simulink model "Spartan2Serial"  (R2019a)
settings: Solver=FixedStepDiscrete  StartTime=0.0  StopTime=inf  FixedStep=0.01  RelTol=1e-3
undefined symbols (not defined in the file): serial
libraries: instrumentlib x2
settings Model: SimulationMode=accelerator  EnablePacing=on  Creator=manuk  LastModifiedBy=manuk
settings DataIOCC: SaveOutput=off  SignalLogging=off  DSMLogging=off  SaveTime=off  ReturnWorkspaceOutputs=off

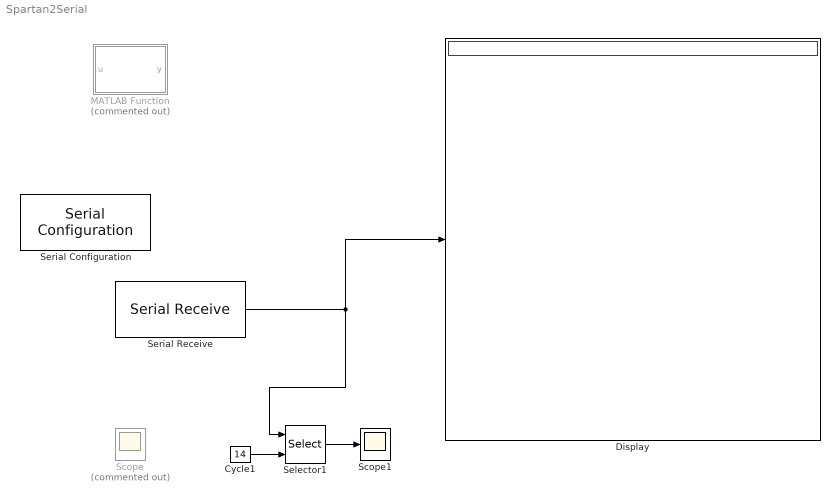
== system Spartan2Serial ==
  Cycle1 : Constant  Value=14
  Display : Display
  MATLAB Function : MATLAB Function  Commented=on  TreatAsAtomicUnit=on
  Scope : Scope  Commented=on
  Scope1 : Scope
  Selector1 : Selector  IndexOptions=Index vector (port)  Indices=[6]  OutputSizes=1
  Serial Configuration : instrumentlib/Serial Configuration  Priority=-200000  ComPortMenu=COM4  ComPort=COM4  ObjConstructor=serial('COM4');  BaudRate=921600  DataBits=8  Parity=none  StopBits=1  FlowControl=none  Timeout=10  ByteOrder=LittleEndian
  Serial Receive : instrumentlib/Serial Receive  ComPortMenu=COM4  ComPort=COM4  ObjConstructor=serial('COM4');  Terminator=<none>  DataSize="[16   1]"  DataType=uint8  EnableBlockingMode=on  ActionDataUnavailable=Output last received value  CustomValue=0  SampleTime=0.01
  wires:
  ? -> Scope/1
  Cycle1/1 -> Selector1/2
  Selector1/1 -> Scope1/1
  Serial Receive/1 -> Display/1, Selector1/1

== matlab function Spartan2Serial/MATLAB Function ==
  data: u input; y output
function y = fcn(u)
coder.extrinsic('fcn');
coder.extrinsic('serial');
coder.extrinsic('fscanf');
s= serial('COM4','BaudRate',115200);
fopen(s);
 a=fscanf(s);
 
flush(s);
fclose(s);
%y=a;
y = u;
